simulink model "sf_4_toy_car"  (R2022b)
settings: Solver=VariableStepAuto  StartTime=0.0  StopTime=50  RelTol=1e-3
settings Model: Creator=user  LastModifiedBy=user

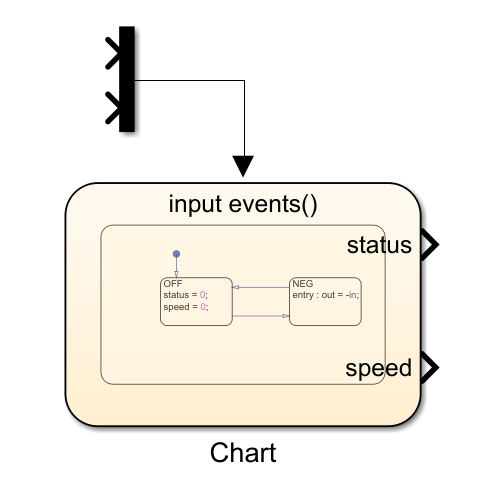
[thumbnail: Simulink's stored preview of the top-level diagram]
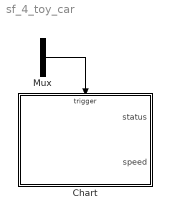
== system sf_4_toy_car ==
  Chart : Stateflow chart  TreatAsAtomicUnit=on
  Mux : Mux  Inputs=2
  wires:
  Mux/1 -> Chart/Trigger

== stateflow chart sf_4_toy_car/Chart ==
  settings: executeAtInitialization=1
  state ?
    state OFF
      status = 0;
      speed = 0;
    state NEG
      entry : out = -in;
    (default) -> OFF
    NEG -> OFF
    OFF -> NEG
  data: status output; speed output
  events: SW input EITHER_EDGE_EVENT; SPD input FUNCTION_CALL_EVENT
